simulink model "rgb2gray_2018b"  (R2018b)
settings: Solver=FixedStepDiscrete  StartTime=0.0  StopTime=totalPixels  RelTol=1e-3
InitFcn:
  | frm2pix = visionhdl.FrameToPixels;
  | frm2pix.VideoFormat = '240p';
  | [activePixelsPerLine, activeLines, totalPixels] = getparamfromfrm2pix(frm2pix);
undefined symbols (not defined in the file): gray, Rec, SDTV, totalPixels
libraries: visionhdlio x2, visionconversions x1, visionsources x1, visionstatistics x1, hdlsllib x1
settings Model: DataTypeOverride=Off  SimulationMode=accelerator  Creator=linbai  LastModifiedBy=lbai
settings DataIOCC: SaveOutput=off  SaveTime=off  ReturnWorkspaceOutputs=on
settings OptimizationCC: BlockReduction=off  ConditionallyExecuteInputs=off  DefaultParameterBehavior=Inlined
settings DebuggingCC: AlgebraicLoopMsg=error  SingleTaskRateTransMsg=error
settings HardwareCC: ProdBitPerPointer=32  ProdBitPerSizeT=32  ProdBitPerPtrDiffT=32  ProdLargestAtomicFloat=None  ProdIntDivRoundTo=Undefined  ProdEndianess=Unspecified  ProdWordSize=32  ProdHWDeviceType=ASIC/FPGA->ASIC/FPGA  TargetBitPerPointer=64  TargetBitPerSizeT=64  TargetBitPerPtrDiffT=64  TargetLongLongMode=on  TargetIntDivRoundTo=Zero  TargetEndianess=LittleEndian  TargetWordSize=64  TargetHWDeviceType=Custom Processor->MATLAB Host Computer  ProdEqTarget=off

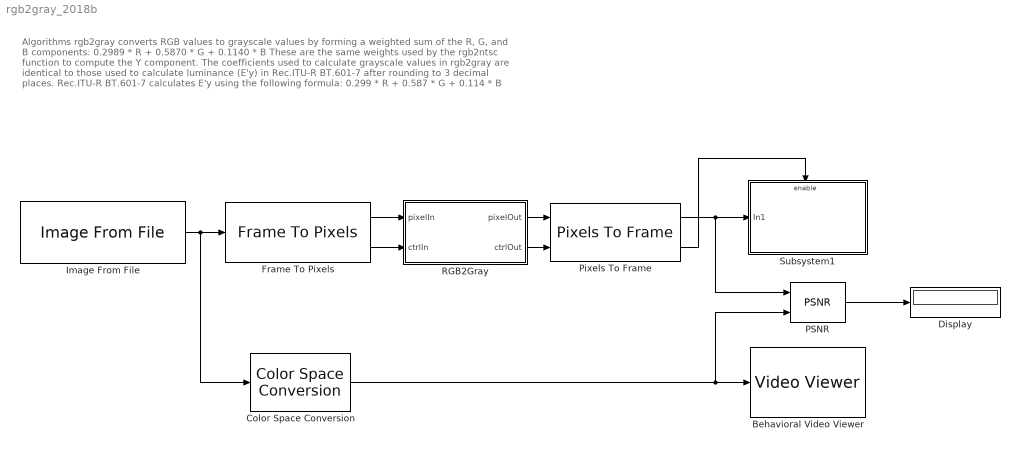
== system rgb2gray_2018b ==
  note: Algorithms
      | rgb2gray converts RGB values to grayscale values by forming a weighted sum of the R, G, and B components:
      | 0.2989 * R + 0.5870 * G + 0.1140 * B
      | These are the same weights used by the rgb2ntsc function to compute the Y component.
      | The coefficients used to calculate grayscale values in rgb2gray are identical to those used to calculate luminance (E'y) in
      | Rec.ITU-R BT.601-7 after rounding to 3 decimal places.
      | Rec.ITU-R BT.601-7 calculates E'y using the following formula:
      | 0.299 * R + 0.587 * G + 0.114 * B
  Behavioral Video Viewer : VideoViewer  colormapValue=gray(256)  FigPos=[166 943 503 381]
  Color Space Conversion : visionconversions/Color Space  Conversion  conversion=Obsolete  conversionActive=R'G'B' to intensity  wp_str=D65  rec=Rec. 601 (SDTV)  sys=1125/60/2:1  imagePorts=One multidimensional signal
  Display : Display
  Frame To Pixels : visionhdlio/Frame To Pixels  NumComponents=3  VideoFormat=240p  ActivePixelsPerLine=160  ActiveVideoLines=160  TotalPixelsPerLine=400  TotalVideoLines=400  StartingActiveLine=6  FrontPorch=120  SampleTime=0
      settings: SourceProductName=Vision HDL Toolbox  SourceProductBaseCode=VT
  Image From File : visionsources/Image From File  Tag=vipblks_nd  FileName=.\img_test_rgb.png  Ts=totalPixels  imagePorts=One multidimensional signal  OutPortLabels=R|G|B  ImageDataType=Inherit from input image  sdImageDataType=uint(8)  Signed=on  WordLength=16  FractionLengthMode=User-defined  FractionLength=15
      settings: SourceProductName=Computer Vision Toolbox
  PSNR : visionstatistics/PSNR
      settings: SourceProductName=Computer Vision Toolbox  SourceProductBaseCode=VP
  Pixels To Frame : visionhdlio/Pixels To Frame  NumComponents=1  VideoFormat=240p  ActivePixelsPerLine=160  ActiveVideoLines=160  TotalPixelsPerLine=400  TotalVideoLines=400
      settings: SourceProductName=Vision HDL Toolbox  SourceProductBaseCode=VT
  RGB2Gray : Subsystem
  Subsystem1 : Subsystem
  wires:
  Image From File/1 -> Color Space Conversion/1, Frame To Pixels/1
  Pixels To Frame/1 -> PSNR/1, Subsystem1/1(In1)
  Pixels To Frame/2 -> Subsystem1/Enable
  Color Space Conversion/1 -> PSNR/2, Behavioral Video Viewer/1
  PSNR/1 -> Display/1
  Frame To Pixels/1 -> RGB2Gray/1(pixelIn)
  Frame To Pixels/2 -> RGB2Gray/2(ctrlIn)
  RGB2Gray/1(pixelOut) -> Pixels To Frame/1
  RGB2Gray/2(ctrlOut) -> Pixels To Frame/2

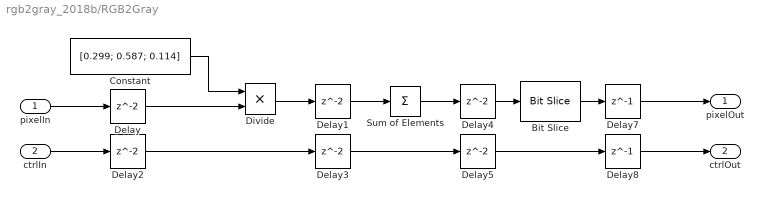
== system rgb2gray_2018b/RGB2Gray ==
  pixelIn : Inport
  ctrlIn : Inport  Port=2
  Bit Slice : hdlsllib/Logic and Bit Operations/Bit Slice  lidx=23  ridx=16
      settings: SourceProductName=Simulink  SourceProductBaseCode=SL
  Constant : Constant  Value=[0.299; 0.587; 0.114]  OutDataTypeStr=fixdt(0,16,16)  SampleTime=-1
  Delay{,1..5} (6 alike) : Delay
  Delay7 : Delay  DelayLength=1
  Delay8 : Delay  DelayLength=1
  Divide : Product  Inputs=**
  Sum of Elements : Sum  Inputs=+
  pixelOut : Outport  VectorParamsAs1DForOutWhenUnconnected=on
  ctrlOut : Outport  Port=2  VectorParamsAs1DForOutWhenUnconnected=on
  wires:
  Constant/1 -> Divide/1
  Divide/1 -> Delay1/1
  Delay5/1 -> Delay8/1
  Delay2/1 -> Delay3/1
  Bit Slice/1 -> Delay7/1
  Delay4/1 -> Bit Slice/1
  Delay/1 -> Divide/2
  Delay1/1 -> Sum of Elements/1
  Sum of Elements/1 -> Delay4/1
  Delay3/1 -> Delay5/1
  pixelIn/1 -> Delay/1
  Delay7/1 -> pixelOut/1
  ctrlIn/1 -> Delay2/1
  Delay8/1 -> ctrlOut/1

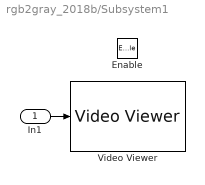
== system rgb2gray_2018b/Subsystem1 ==
  In1 : Inport
  Enable : EnablePort
  Video Viewer : VideoViewer  colormapValue=gray(256)  FigPos=[207 554 441 346]
  wires:
  In1/1 -> Video Viewer/1
